simulink model "power_active_filter_mpc"  (R2019a)
settings: Solver=VariableStepAuto  StartTime=0.0  StopTime=1.5  RelTol=1e-3
values from neighbouring files (symbols this model uses):
  Ts = 2e-6    (= 2e-06)    [parameters.m]
  Vdc = AF.activefilter.voltage    [parameters.m]
undefined symbols (not defined in the file or in its folder): AF, D1, Delta, R
libraries: powerlib x28, powerlib_meascontrol x4, eeTransforms x3, dspstat3 x2, dsparch4 x2, simulink x1, eePwmGeneratorTwoLevel x1
settings Model: PauseTimes=0.51  Creator=Abdullah  LastModifiedBy=Abdullah
settings SolverCC: ShapePreserveControl=EnableAll  MinimalZcImpactIntegration=on
settings DataIOCC: SaveFormat=StructureWithTime  ReturnWorkspaceOutputs=off
settings DebuggingCC: ReadBeforeWriteMsg=DisableAll  WriteAfterWriteMsg=DisableAll  WriteAfterReadMsg=DisableAll  MultiTaskDSMMsg=none
settings ModelReferenceCC: UpdateModelReferenceTargets=IfOutOfDate
settings SFSimCC: SFSimEcho=off

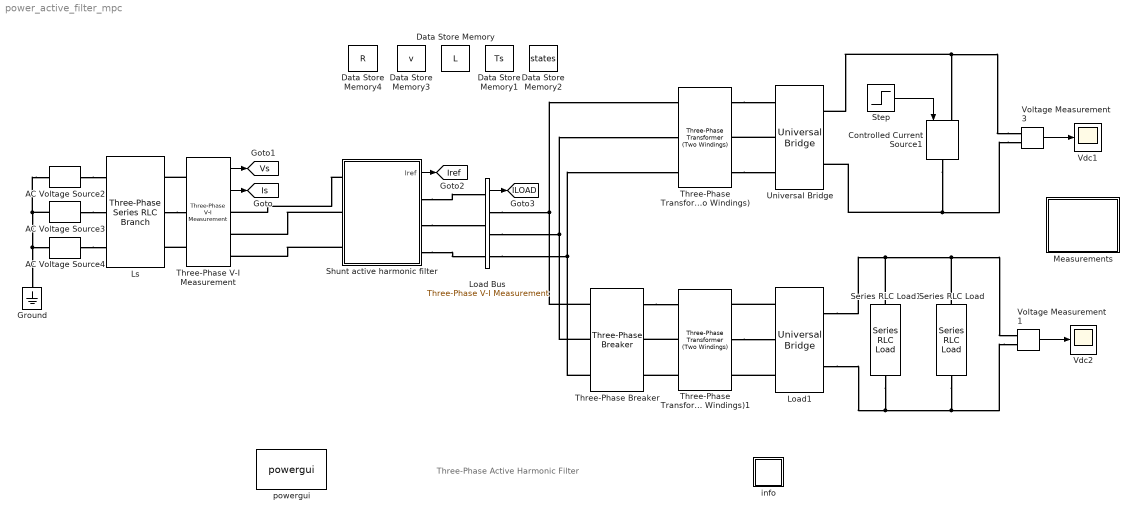
== system power_active_filter_mpc ==
  note: Three-Phase Active Harmonic Filter
  AC Voltage Source2 : powerlib/Electrical Sources/AC Voltage Source  Amplitude=380*sqrt(2)/sqrt(3)  Phase=0  Frequency=50  SampleTime=0  Measurements=None  BusType=swing  Pref=10e3  Qref=0  Qmin=-inf  Qmax=+inf
      settings: SourceProductName=Simscape Electrical
  AC Voltage Source3 : powerlib/Electrical Sources/AC Voltage Source  Amplitude=380*sqrt(2)/sqrt(3)  Phase=-120  Frequency=50  SampleTime=0  Measurements=None  BusType=swing  Pref=10e3  Qref=0  Qmin=-inf  Qmax=+inf
      settings: SourceProductName=Simscape Electrical
  AC Voltage Source4 : powerlib/Electrical Sources/AC Voltage Source  Amplitude=380*sqrt(2)/sqrt(3)  Phase=120  Frequency=50  SampleTime=0  Measurements=None  BusType=swing  Pref=10e3  Qref=0  Qmin=-inf  Qmax=+inf
      settings: SourceProductName=Simscape Electrical
  Controlled Current Source1 : powerlib/Electrical Sources/Controlled Current Source  Initialize=on  Source_Type=AC  Amplitude=0  Phase=0  Frequency=0  Measurements=None
      settings: SourceProductName=Simscape Electrical
  Data Store Memory : DataStoreMemory  DataStoreName=L  ReadBeforeWriteMsg=warning  WriteAfterWriteMsg=warning  WriteAfterReadMsg=warning  InitialValue=L  ShowAdditionalParam=off  OutDataTypeStr=double
  Data Store Memory1 : DataStoreMemory  DataStoreName=Ts  ReadBeforeWriteMsg=warning  WriteAfterWriteMsg=warning  WriteAfterReadMsg=warning  InitialValue=Ts  ShowAdditionalParam=off  OutDataTypeStr=double
  Data Store Memory2 : DataStoreMemory  DataStoreName=states  ReadBeforeWriteMsg=warning  WriteAfterWriteMsg=warning  WriteAfterReadMsg=warning  InitialValue=states  VectorParams1D=off  ShowAdditionalParam=off  OutDataTypeStr=double
  Data Store Memory3 : DataStoreMemory  DataStoreName=v  ReadBeforeWriteMsg=warning  WriteAfterWriteMsg=warning  WriteAfterReadMsg=warning  InitialValue=v  ShowAdditionalParam=off  OutDataTypeStr=double
      settings: SignalType=complex
  Data Store Memory4 : DataStoreMemory  DataStoreName=R  ReadBeforeWriteMsg=warning  WriteAfterWriteMsg=warning  WriteAfterReadMsg=warning  InitialValue=R  ShowAdditionalParam=off  OutDataTypeStr=double
  Ground : powerlib/Elements/Ground  LConnTagsString=a
      settings: SourceProductName=Simscape Electrical
  Load Bus : powerlib/Measurements/Three-Phase V-I Measurement  VoltageMeasurement=no  SetLabelV=off  LabelV=Vabc  Vpu=off  VpuLL=off  CurrentMeasurement=yes  SetLabelI=off  LabelI=ILoad  Ipu=off  Pbase=100e6  Vbase=500e3  OutputType=Complex  PhasorSimulation=off  PSBequivalent=0
      settings: SourceProductName=Simscape Electrical
  Load1 : powerlib/Power Electronics/Universal Bridge  Arms=3  SnubberResistance=1e3  SnubberCapacitance=1e-6  Device=Diodes  Ron=1e-3  Lon=0  ForwardVoltages="[  0  0  ]"  ForwardVoltage=0  GTOparameters=[ 10e-6 , 20e-6 ]  IGBTparameters=[ 1e-6 , 2e-6 ]  Measurements=None  Measurements_2=None  converterType=Rectifier
      settings: SourceProductName=Simscape Electrical
  Ls : powerlib/Elements/Three-Phase Series RLC Branch  LConnTagsString=A|B|C  RConnTagsString=A|B|C  BranchType=L  Resistance=1  Inductance=1e-5  Capacitance=1e-6  Measurements=None
      settings: SourceProductName=Simscape Electrical
  Measurements : Subsystem
  Series RLC Load : powerlib/Elements/Series RLC Load  LConnTagsString=a  RConnTagsString=__new0  NominalVoltage=500  NominalFrequency=50  ActivePower=50e3  InductivePower=10e3  CapacitivePower=0  Setx0=off  InitialVoltage=0  SetiL0=off  InitialCurrent=0  Measurements=None  LoadType=constant Z
      settings: SourceProductName=Simscape Electrical
  Series RLC Load1 : powerlib/Elements/Series RLC Load  LConnTagsString=a  RConnTagsString=__new0  NominalVoltage=500  NominalFrequency=50  ActivePower=0  InductivePower=0  CapacitivePower=20e3  Setx0=off  InitialVoltage=0  SetiL0=off  InitialCurrent=0  Measurements=None  LoadType=constant Z
      settings: SourceProductName=Simscape Electrical
  Shunt active harmonic filter : Subsystem  mask(Parallel Active Filter){platform=AF}
  Step : Step  Time=0.5  Before=100  After=160  SampleTime=0
  Three-Phase Transformer (Two Windings) : powerlib/Elements/Three-Phase Transformer (Two Windings)  Winding1Connection=Delta (D1)  Winding2Connection=Delta (D1)  CoreType=Three single-phase transformers  SetSaturation=off  Hysteresis=off  DataFile='hysteresis'  SetInitialFlux=off  Measurements=None  UNITS=pu  NominalPower=[ 500e3 , 50 ]  Winding1=[380, 0.002 , 0.08 ]  Winding2=[380, 0.002 , 0.08 ]  Rm=500  Lm=500  L0=0.5  Saturation=[ 0,0 ; 0.0024,1.2 ; 1.0,1.52 ]  InitialFluxes=[ 0.8 , -0.8 , 0.7 ]  BreakLoop=off  DiscreteSolver=Trapezoidal iterative  DataType=off  TransfoNumber=0
      settings: SourceProductName=Simscape Electrical
  Three-Phase Transformer (Two Windings)1 : powerlib/Elements/Three-Phase Transformer (Two Windings)  Winding1Connection=Delta (D1)  Winding2Connection=Y  CoreType=Three single-phase transformers  SetSaturation=off  Hysteresis=off  DataFile='hysteresis'  SetInitialFlux=off  Measurements=None  UNITS=pu  NominalPower=[ 500e3 , 50 ]  Winding1=[380, 0.002 , 0.08 ]  Winding2=[380, 0.002 , 0.08 ]  Rm=500  Lm=500  L0=0.5  Saturation=[ 0,0 ; 0.0024,1.2 ; 1.0,1.52 ]  InitialFluxes=[-0.000126716792896904 1.12530200800683e-05 0.000115463772816653]  BreakLoop=off  DiscreteSolver=Trapezoidal iterative  DataType=off  TransfoNumber=0
      settings: SourceProductName=Simscape Electrical
  Three-Phase V-I Measurement : powerlib/Measurements/Three-Phase V-I Measurement  VoltageMeasurement=phase-to-ground  SetLabelV=off  LabelV=Vabc  Vpu=off  VpuLL=off  CurrentMeasurement=yes  SetLabelI=off  LabelI=Iabc  Ipu=off  Pbase=100e6  Vbase=500e3  OutputType=Complex  PhasorSimulation=off  PSBequivalent=0
      settings: SourceProductName=Simscape Electrical
  Three-Phase Breaker : powerlib/Elements/Three-Phase Breaker  InitialState=open  SwitchA=on  SwitchB=on  SwitchC=on  SwitchTimes=1  External=off  BreakerResistance=1e-5  SnubberResistance=1e6  SnubberCapacitance=inf  Measurements=None
      settings: SourceProductName=Simscape Electrical
  Universal Bridge : powerlib/Power Electronics/Universal Bridge  Arms=3  SnubberResistance=1e5  SnubberCapacitance=inf  Device=Diodes  Ron=1e-3  Lon=0  ForwardVoltages="[  0  0  ]"  ForwardVoltage=0  GTOparameters=[ 10e-6 , 20e-6 ]  IGBTparameters=[ 1e-6 , 2e-6 ]  Measurements=None  Measurements_2=None  converterType=Rectifier
      settings: SourceProductName=Simscape Electrical
  Vdc1 : Scope
  Vdc2 : Scope
  Voltage Measurement1 : powerlib/Measurements/Voltage Measurement  PhasorSimulation=off  OutputType=Complex  PSBequivalent=0
      settings: SourceProductName=Simscape Electrical
  Voltage Measurement3 : powerlib/Measurements/Voltage Measurement  PhasorSimulation=off  OutputType=Complex  PSBequivalent=0
      settings: SourceProductName=Simscape Electrical
  info : Subsystem
      settings: OpenFcn=showdemo(bdroot(gcb))
      mask Display: disp('?')
  powergui : powerlib/powergui  SimulationMode=Discrete  SampleTime=Ts  frequency=60  Iterations=50  frequencyindice=0  Pbase=100e6  ErrMax=1e-4  UnitsV=kV  UnitsW=MW  buscounter=0  FunctionMessages=off  echomessages=off  EnableUseOfTLC=off  CurrentSourceSwitches=off  DisableSnubberDevices=off  DisableRonSwitches=off  DisableVfSwitches=off  DisplayEquations=off  AutomaticDiscreteSolvers=off  SolverType=Tustin/Backward Euler (TBE)  Interpol=off  ExternalGateDelay=off  methode=off  Ts=0  x0status=blocks  SPID=off  SwTol=0  HookPort=off  NonlinearTolerance=0  nMaxIteration=15  ContinueOnMaxIteration=off  RestoreLinks=warning  ResistiveCurrentMeasurement=off  Frange=[0:2:500]  Ylog=off  Xlog=on  ShowGrid=off  save=off  variable=ZData  structure=Filteroutput  ZoomFFT=off  StartTime=10/50  cycles=2  DisplayStyle=1  fundamental=50  FreqAxis=on  MaxFrequency=250000  frequencyindicesteady=1  RmsSteady=1  display=off
      settings: SourceProductName=Simscape Electrical
  tag scope: ILOAD=global, Iref=global, Is=global, Vs=global
  wires:
  Load Bus/1 -> [ILOAD]
  Three-Phase V-I Measurement/1 -> [Vs]
  Voltage Measurement3/1 -> Vdc1/1
  Shunt active harmonic filter/1(Iref) -> [Iref]
  Step/1 -> Controlled Current Source1/1
  Three-Phase V-I Measurement/2 -> [Is]
  Voltage Measurement1/1 -> Vdc2/1
  connections:
  Load Bus/RConn3 -- Three-Phase Breaker/LConn3 -- Three-Phase Transformer (Two Windings)/LConn3
  Load Bus/RConn1 -- Three-Phase Breaker/LConn1 -- Three-Phase Transformer (Two Windings)/LConn1
  Voltage Measurement3/LConn2 -- Universal Bridge/RConn2 -- Controlled Current Source1/RConn1
  AC Voltage Source2/LConn1 -- AC Voltage Source4/LConn1 -- Ground/LConn1 -- AC Voltage Source3/LConn1
  Load Bus/RConn2 -- Three-Phase Breaker/LConn2 -- Three-Phase Transformer (Two Windings)/LConn2
  Series RLC Load1/LConn1 -- Load1/RConn1 -- Series RLC Load/LConn1 -- Voltage Measurement1/LConn1
  Voltage Measurement1/LConn2 -- Series RLC Load/RConn1 -- Load1/RConn2 -- Series RLC Load1/RConn1
  Voltage Measurement3/LConn1 -- Universal Bridge/RConn1 -- Controlled Current Source1/LConn1
  AC Voltage Source4/RConn1 -- Ls/LConn3
  Shunt active harmonic filter/LConn3 -- Three-Phase V-I Measurement/RConn3
  Shunt active harmonic filter/LConn2 -- Three-Phase V-I Measurement/RConn2
  Three-Phase Transformer (Two Windings)/RConn1 -- Universal Bridge/LConn1
  Shunt active harmonic filter/RConn3 -- Load Bus/LConn3
  Shunt active harmonic filter/RConn1 -- Load Bus/LConn1
  Shunt active harmonic filter/RConn2 -- Load Bus/LConn2
  Shunt active harmonic filter/LConn1 -- Three-Phase V-I Measurement/RConn1
  Universal Bridge/LConn2 -- Three-Phase Transformer (Two Windings)/RConn2
  Three-Phase V-I Measurement/LConn1 -- Ls/RConn1
  Ls/RConn2 -- Three-Phase V-I Measurement/LConn2
  Three-Phase V-I Measurement/LConn3 -- Ls/RConn3
  AC Voltage Source2/RConn1 -- Ls/LConn1
  AC Voltage Source3/RConn1 -- Ls/LConn2
  Three-Phase Transformer (Two Windings)/RConn3 -- Universal Bridge/LConn3
  Load1/LConn1 -- Three-Phase Transformer (Two Windings)1/RConn1
  Three-Phase Transformer (Two Windings)1/RConn2 -- Load1/LConn2
  Load1/LConn3 -- Three-Phase Transformer (Two Windings)1/RConn3
  Three-Phase Breaker/RConn1 -- Three-Phase Transformer (Two Windings)1/LConn1
  Three-Phase Transformer (Two Windings)1/LConn2 -- Three-Phase Breaker/RConn2
  Three-Phase Transformer (Two Windings)1/LConn3 -- Three-Phase Breaker/RConn3

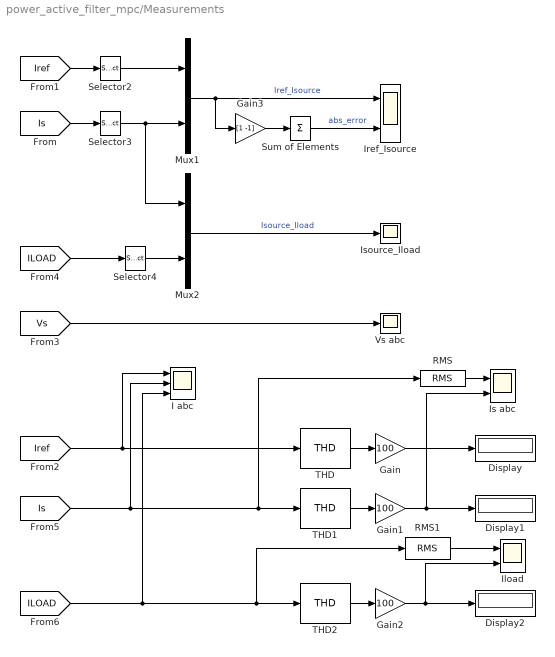
== system power_active_filter_mpc/Measurements ==
  Display : Display
  Display1 : Display
      settings: Decimation=2
  Display2 : Display
      settings: Decimation=2
  Gain : Gain  Gain=100
  Gain1 : Gain  Gain=100
  Gain2 : Gain  Gain=100
  Gain3 : Gain  Gain=[1 -1]
  I abc : Scope  NumInputPorts=3
  Iload : Scope  NumInputPorts=2
  Iref_Isource : Scope  NumInputPorts=2
  Is abc : Scope  NumInputPorts=2
  Isource_Iload : Scope
  Mux1 : Mux  Inputs=2
  Mux2 : Mux  Inputs=2
  RMS : dspstat3/RMS  run=off  directionMode=Each column  dimension=1  InputProcessing=Columns as channels (frame based)  reset_popup=None
  RMS1 : dspstat3/RMS  run=off  directionMode=Each column  dimension=1  InputProcessing=Columns as channels (frame based)  reset_popup=None
  Selector2 : Selector  InputPortWidth=3  IndexOptions=Index vector (dialog)  Indices=1  OutputSizes=1
  Selector3 : Selector  InputPortWidth=3  IndexOptions=Index vector (dialog)  Indices=1  OutputSizes=1
  Selector4 : Selector  InputPortWidth=3  IndexOptions=Index vector (dialog)  Indices=1  OutputSizes=1
  Sum of Elements : Sum  Inputs=+
  THD : powerlib_meascontrol/Measurements/THD  Freq=50  Ts=0
      settings: SourceProductName=Simscape Electrical
  THD1 : powerlib_meascontrol/Measurements/THD  Freq=50  Ts=0
      settings: SourceProductName=Simscape Electrical
  THD2 : powerlib_meascontrol/Measurements/THD  Freq=50  Ts=0
      settings: SourceProductName=Simscape Electrical
  Vs abc : Scope
  wires:
  Mux1/1 -> Gain3/1, Iref_Isource/1  "Iref_Isource"
  Selector2/1 -> Mux1/1
  Selector3/1 -> Mux1/2, Mux2/1
  [Iref] -> Selector2/1
  [Is] -> Selector3/1
  Mux2/1 -> Isource_Iload/1  "Isource_Iload"
  Selector4/1 -> Mux2/2
  [ILOAD] -> Selector4/1
  Gain3/1 -> Sum of Elements/1
  Sum of Elements/1 -> Iref_Isource/2  "abs_error"
  [Vs] -> Vs abc/1
  [Iref] -> THD/1, I abc/1
  [Is] -> RMS/1, THD1/1, I abc/2
  THD/1 -> Gain/1
  THD1/1 -> Gain1/1
  Gain/1 -> Display/1
  Gain1/1 -> Is abc/2, Display1/1
  THD2/1 -> Gain2/1
  RMS/1 -> Is abc/1
  RMS1/1 -> Iload/1
  Gain2/1 -> Iload/2, Display2/1
  [ILOAD] -> I abc/3, RMS1/1, THD2/1

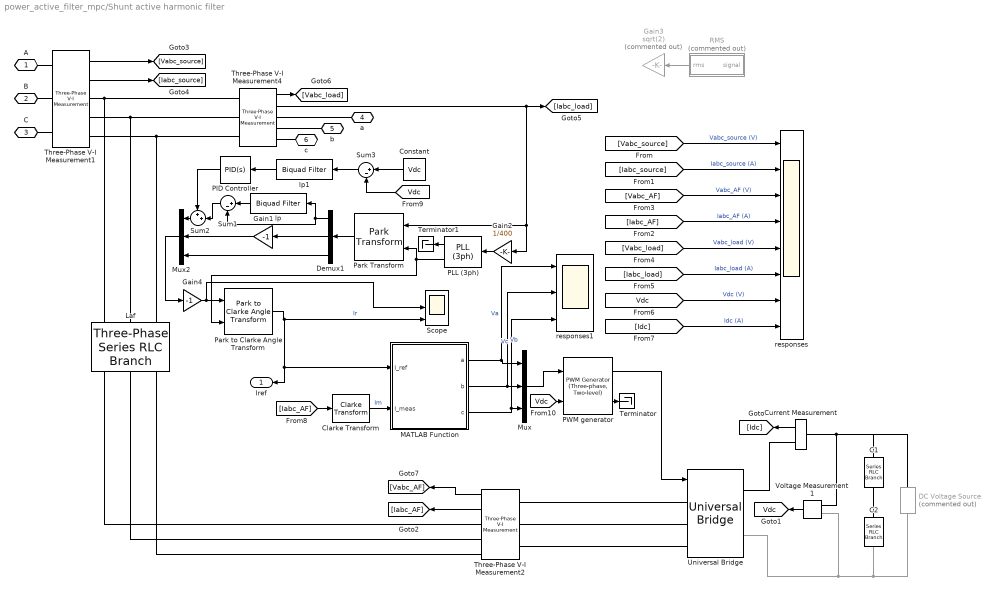
== system power_active_filter_mpc/Shunt active harmonic filter ==
  C1 : powerlib/Elements/Series RLC Branch  LConnTagsString=__new0  RConnTagsString=__new0  BranchType=C  Resistance=1  Inductance=1e-3  SetiL0=off  InitialCurrent=0  Capacitance=platform.activefilter.DC_cap  Setx0=on  InitialVoltage=Vdc/2  Measurements=None
      settings: SourceProductName=Simscape Electrical
  C2 : powerlib/Elements/Series RLC Branch  LConnTagsString=__new0  RConnTagsString=__new0  BranchType=C  Resistance=1  Inductance=1e-3  SetiL0=off  InitialCurrent=0  Capacitance=platform.activefilter.DC_cap  Setx0=on  InitialVoltage=Vdc/2  Measurements=None
      settings: SourceProductName=Simscape Electrical
  Clarke Transform : eeTransforms/Clarke Transform  PowerInvariant=off
      settings: SourceProductName=Simscape Electrical  SourceProductBaseCode=PS
  Constant : Constant  Value=Vdc
  Current Measurement : powerlib/Measurements/Current Measurement  PhasorSimulation=off  OutputType=Complex  PSBequivalent=0
      settings: SourceProductName=Simscape Electrical
  DC Voltage Source : powerlib/Electrical Sources/DC Voltage Source  Commented=on  Amplitude=Vdc  Measurements=None
      settings: SourceProductName=Simscape Electrical
  Demux1 : Demux  Outputs=3
  Gain1 : Gain  Gain=-1
  Gain2 : Gain  Gain=1/400
  Gain3 : Gain  Commented=on  Gain=sqrt(2)
  Gain4 : Gain  Gain=-1
  Laf : powerlib/Elements/Three-Phase Series RLC Branch  LConnTagsString=A|B|C  RConnTagsString=A|B|C  BranchType=RL  Resistance=R  Inductance=platform.activefilter.Laf  Capacitance=1e-6  Measurements=None
      settings: SourceProductName=Simscape Electrical
  MATLAB Function : MATLAB Function  TreatAsAtomicUnit=on  SystemSampleTime=Ts
  Mux : Mux  Inputs=3
  Mux2 : Mux  Inputs=3
  PID Controller : simulink/Continuous/PID Controller  Controller=PID  Form=Parallel  TimeDomain=Continuous-time  SampleTime=-1  IntegratorMethod=Forward Euler  FilterMethod=Forward Euler  ControllerParametersSource=internal  P=0.0255  I=0.75  D=0.0005  UseFilter=on  N=100  TunerSelectOption=Transfer Function Based (PID Tuner App)  InitialConditionSource=internal  InitialConditionForIntegrator=0  InitialConditionForFilter=0  DifferentiatorICPrevScaledInput=0  ExternalReset=none  TrackingMode=off  Kt=1  LimitOutput=off  UpperSaturationLimit=inf  LowerSaturationLimit=-inf  LinearizeAsGain=on  AntiWindupMode=none  Kb=1  POutMin=[]  POutMax=[]  IOutMin=[]  IOutMax=[]  DOutMin=[]  DOutMax=[]  NOutMin=[]  NOutMax=[]  SumOutMin=[]  SumOutMax=[]  SaturationOutMin=[]  SaturationOutMax=[]  PParamMin=[]  PParamMax=[]  IParamMin=[]  IParamMax=[]  DParamMin=[]  DParamMax=[]  NParamMin=[]  NParamMax=[]  KbParamMin=[]  KbParamMax=[]  KtParamMin=[]  KtParamMax=[]  KbOutMin=[]  KbOutMax=[]  KtOutMin=[]  KtOutMax=[]  IntegratorOutMin=[]  IntegratorOutMax=[]  FilterOutMin=[]  FilterOutMax=[]  SumI1OutMin=[]  SumI1OutMax=[]  SumI2OutMin=[]  SumI2OutMax=[]  SumI3OutMin=[]  SumI3OutMax=[]  SumI4OutMin=[]  SumI4OutMax=[]  SumDOutMin=[]  SumDOutMax=[]  DifferentiatorOutMin=[]  DifferentiatorOutMax=[]  FilterDiffOutCoefMin=[]  FilterDiffOutCoefMax=[]  ReciprocalOutMin=[]  ReciprocalOutMax=[]  SumDenOutMin=[]  SumDenOutMax=[]  SumNumOutMin=[]  SumNumOutMax=[]  DivideOutMin=[]  DivideOutMax=[]  IntegratorContinuousStateAttributes=''  IntegratorStateMustResolveToSignalObject=off  IntegratorRTWStateStorageClass=Auto  FilterContinuousStateAttributes=''  FilterStateMustResolveToSignalObject=off  FilterRTWStateStorageClass=Auto  ParallelPVariant=InternalParameters  IdealPVariant=Disabled  IVariant=InternalParameters  DVariant=InternalParameters  IntegratorVariant=Continuous  SatVariant=Disabled  AWVariant=Passthrough  PCopyVariant=Disabled  TRVariant=Disabled  FdbkBlocksVariant=Forward  IdealPFdbkVariant=Disabled  SatFdbkVariant=Disabled  DerivativeFilterVariant=ContFilter  NVariant=InternalParameters  NCopyVariant=Disabled  FilterICVariant=InternalICsFilter  IntegratorICVariant=InternalICs  ExternalResetVariant=Disabled  TRSumVariant=Passthrough  SumFdbkVariant=Disabled  SumVariant=Sum_PID
  PLL (3ph) : powerlib_meascontrol/PLL/PLL (3ph)  Fmin=45  Par_Init=[0 50]  ParK=[ 180 3200 1 ]  TcD=1e-3  MaxRateChangeFreq=12  FilterCutOffFreq=25  Ts=Ts  AGC=on
      settings: SourceProductName=Simscape Electrical
  PWM generator : eePwmGeneratorTwoLevel/PWM Generator (Three-phase, Two-level)  PWMMode=Continuous PWM (CPWM)  CPWMMode=SPWM: sinusoidal PWM  DPWMMode=60 DPWM: 60 degree discontinuous PWM  fsw=5000  Ts=Ts
      settings: SourceProductName=Simscape Electrical  SourceProductBaseCode=PS
  Park Transform : eeTransforms/Park Transform  AxisAlignment=Q-axis  PowerInvariant=off
      settings: SourceProductName=Simscape Electrical
  Park to Clarke Angle Transform : eeTransforms/Park to Clarke Angle Transform  AxisAlignment=Q-axis
      settings: SourceProductName=Simscape Electrical  SourceProductBaseCode=PS
  RMS : Subsystem  Commented=on  DialogController=POWERSYS.PowerSysDialog  mask(RMS){f1=platform.activefilter.freq}
      mask prompts: f1 "Fundamental frequency (Hz):"
      mask help: This block measures the root mean square value of instantaneous current or voltage signal connected to the input of the block. The RMS value is calculated over a running window of one cycle of the specified fundamental frequency.
      mask init:
      | power_initmask();
      mask Help: helpview(psbhelp)
  Scope : Scope  NumInputPorts=3
  Sum1 : Sum  Inputs=|+-
  Sum2 : Sum  Inputs=++|
  Sum3 : Sum  Inputs=|+-
  Terminator : Terminator
  Terminator1 : Terminator
  Three-Phase V-I Measurement1 : powerlib/Measurements/Three-Phase V-I Measurement  VoltageMeasurement=phase-to-phase  SetLabelV=off  LabelV=Vabc  Vpu=off  VpuLL=off  CurrentMeasurement=yes  SetLabelI=off  LabelI=Iabc  Ipu=off  Pbase=100e6  Vbase=500e3  OutputType=Complex  PhasorSimulation=off  PSBequivalent=0
      settings: SourceProductName=Simscape Electrical
  Three-Phase V-I Measurement2 : powerlib/Measurements/Three-Phase V-I Measurement  VoltageMeasurement=phase-to-phase  SetLabelV=off  LabelV=Vabc  Vpu=off  VpuLL=off  CurrentMeasurement=yes  SetLabelI=off  LabelI=Iabc  Ipu=off  Pbase=100e6  Vbase=500e3  OutputType=Complex  PhasorSimulation=off  PSBequivalent=0
      settings: SourceProductName=Simscape Electrical
  Three-Phase V-I Measurement4 : powerlib/Measurements/Three-Phase V-I Measurement  VoltageMeasurement=phase-to-phase  SetLabelV=off  LabelV=Vabc  Vpu=off  VpuLL=off  CurrentMeasurement=yes  SetLabelI=off  LabelI=Iabc  Ipu=off  Pbase=100e6  Vbase=500e3  OutputType=Complex  PhasorSimulation=off  PSBequivalent=0
      settings: SourceProductName=Simscape Electrical
  Universal Bridge : powerlib/Power Electronics/Universal Bridge  Arms=3  SnubberResistance=1e5  SnubberCapacitance=inf  Device=IGBT / Diodes  Ron=1e-3  Lon=0  ForwardVoltages="[  0  0  ]"  ForwardVoltage=0  GTOparameters=[ 10e-6 , 20e-6 ]  IGBTparameters=[ 1e-6 , 2e-6 ]  Measurements=None  Measurements_2=None  converterType=Rectifier
      settings: SourceProductName=Simscape Electrical
  Voltage Measurement1 : powerlib/Measurements/Voltage Measurement  PhasorSimulation=off  OutputType=Complex  PSBequivalent=0
      settings: SourceProductName=Simscape Electrical
  lp : dsparch4/Biquad Filter  Tag=BlockMethodSubSystem  FilterSource=Dialog parameters  CoeffSource=Specify via dialog  FilterObject=BQF  IIRFiltStruct=Direct form II  BiQuadCoeffs=[0.0548343892941136057 -0.109665070395729369 0.0548343892941136266 1 -1.99845906585976141 0.998464270664409792;1.00001025426045609 -2 1.00001025426045587 1 -1.99980794984853238 0.999822128007448074;0.00102649751294326286 0.00102649751294326286 0 1 -0.998953802933608026 0;1.00001336148623721 -2 1.00001336148623721 1 -1.99929745179046936 0.999308704544053739]  ScaleValues=[3.31889887857111711e-06;1;1;1;62738.3781479644313]  IC=0  ICnum=0  ICden=0  a0Flag=Warning  optimizeScaleValues=on  ScaleValueMode=Specify via input port (g)  roundingMode=Floor  overflowMode=off  scaleValueFracLength=14  denProdOutputFracLength=30  denAccumFracLength=30  secondMemoryFracLength=15
      settings: SourceProductName=DSP System Toolbox
  lp1 : dsparch4/Biquad Filter  Tag=BlockMethodSubSystem  FilterSource=Dialog parameters  CoeffSource=Specify via dialog  FilterObject=BQF  IIRFiltStruct=Direct form II  BiQuadCoeffs=[0.0548343892941136057 -0.109665070395729369 0.0548343892941136266 1 -1.99845906585976141 0.998464270664409792;1.00001025426045609 -2 1.00001025426045587 1 -1.99980794984853238 0.999822128007448074;0.00102649751294326286 0.00102649751294326286 0 1 -0.998953802933608026 0;1.00001336148623721 -2 1.00001336148623721 1 -1.99929745179046936 0.999308704544053739]  ScaleValues=[3.31889887857111711e-06;1;1;1;62738.3781479644313]  IC=0  ICnum=0  ICden=0  a0Flag=Warning  optimizeScaleValues=on  ScaleValueMode=Specify via input port (g)  roundingMode=Floor  overflowMode=off  scaleValueFracLength=14  denProdOutputFracLength=30  denAccumFracLength=30  secondMemoryFracLength=15
      settings: SourceProductName=DSP System Toolbox
  responses : Scope  NumInputPorts=8
  responses1 : Scope  NumInputPorts=3
  A : PMIOPort  Side=Left
  B : PMIOPort  Port=2  Side=Left
  C : PMIOPort  Port=3  Side=Left
  a : PMIOPort  Port=4  Side=Right
  b : PMIOPort  Port=5  Side=Right
  c : PMIOPort  Port=6  Side=Right
  Iref : Outport
  tag scope: Vdc=global
  wires:
  Three-Phase V-I Measurement2/2 -> [Iabc_AF]
  Current Measurement/1 -> [Idc]
  RMS/1(rms) -> Gain3/1
  Voltage Measurement1/1 -> [Vdc]
  Three-Phase V-I Measurement2/1 -> [Vabc_AF]
  Three-Phase V-I Measurement4/1 -> [Vabc_load]
  Three-Phase V-I Measurement1/1 -> [Vabc_source]
  Three-Phase V-I Measurement1/2 -> [Iabc_source]
  [Vabc_source] -> responses/1  "Vabc_source (V)"
  [Iabc_source] -> responses/2  "Iabc_source (A)"
  [Vabc_AF] -> responses/3  "Vabc_AF (V)"
  [Iabc_AF] -> responses/4  "Iabc_AF (A)"
  [Vabc_load] -> responses/5  "Vabc_load (V)"
  [Iabc_load] -> responses/6  "Iabc_load (A)"
  [Vdc] -> responses/7  "Vdc (V)"
  [Idc] -> responses/8  "Idc (A)"
  Clarke Transform/1 -> MATLAB Function/2(I_meas)  "Im"
  [Iabc_AF] -> Clarke Transform/1
  Gain2/1 -> PLL (3ph)/1
  PLL (3ph)/2 -> Park Transform/2, Park to Clarke Angle Transform/2
  Three-Phase V-I Measurement4/2 -> [Iabc_load], Park Transform/1, Gain2/1
  Park Transform/1 -> Demux1/1
  Demux1/1 -> Sum1/2, lp/1
  Demux1/3 -> Mux2/3
  lp/1 -> Sum1/1
  Demux1/2 -> Gain1/1
  Park to Clarke Angle Transform/1 -> Scope/3, MATLAB Function/1(I_ref), Iref/1  "Ir"
  Gain1/1 -> Mux2/2
  Gain4/1 -> Scope/2, Park to Clarke Angle Transform/1
  Mux2/1 -> Gain4/1
  Constant/1 -> Sum3/1
  [Vdc] -> Sum3/2
  Sum3/1 -> lp1/1
  lp1/1 -> PID Controller/1
  PID Controller/1 -> Sum2/1
  [Vdc] -> PWM generator/2
  Mux/1 -> PWM generator/1
  PWM generator/2 -> Terminator/1
  PLL (3ph)/1 -> Terminator1/1
  MATLAB Function/2(b) -> responses1/2, Mux/2  "Vb"
  MATLAB Function/1(a) -> responses1/1, Mux/1  "Va"
  MATLAB Function/3(c) -> responses1/3, Mux/3  "Vc"
  PWM generator/1 -> Universal Bridge/1
  Sum2/1 -> Mux2/1
  Sum1/1 -> Sum2/2
  connections:
  Voltage Measurement1/LConn1 -- C1/LConn1 -- DC Voltage Source/RConn1 -- Current Measurement/LConn1
  C2/LConn1 -- C1/RConn1
  DC Voltage Source/LConn1 -- C2/RConn1 -- Universal Bridge/RConn2 -- Voltage Measurement1/LConn2
  Universal Bridge/RConn1 -- Current Measurement/RConn1
  Three-Phase V-I Measurement1/RConn1 -- Three-Phase V-I Measurement4/LConn1 -- Laf/RConn1
  Three-Phase V-I Measurement1/RConn2 -- Three-Phase V-I Measurement4/LConn2 -- Laf/RConn2
  Three-Phase V-I Measurement1/RConn3 -- Three-Phase V-I Measurement4/LConn3 -- Laf/RConn3
  a/RConn1 -- Three-Phase V-I Measurement4/RConn1
  b/RConn1 -- Three-Phase V-I Measurement4/RConn2
  c/RConn1 -- Three-Phase V-I Measurement4/RConn3
  C/RConn1 -- Three-Phase V-I Measurement1/LConn3
  Three-Phase V-I Measurement1/LConn2 -- B/RConn1
  A/RConn1 -- Three-Phase V-I Measurement1/LConn1
  Three-Phase V-I Measurement2/LConn2 -- Universal Bridge/LConn2
  Universal Bridge/LConn1 -- Three-Phase V-I Measurement2/LConn1
  Three-Phase V-I Measurement2/LConn3 -- Universal Bridge/LConn3
  Three-Phase V-I Measurement2/RConn3 -- Laf/LConn3
  Three-Phase V-I Measurement2/RConn2 -- Laf/LConn2
  Three-Phase V-I Measurement2/RConn1 -- Laf/LConn1

== system power_active_filter_mpc/info ==

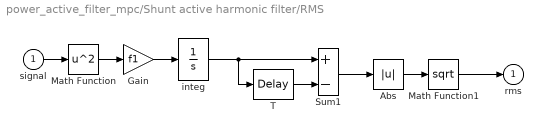
== system power_active_filter_mpc/Shunt active harmonic filter/RMS ==
  signal : Inport
  Abs : Abs  SaturateOnIntegerOverflow=on
  Gain : Gain  Gain=f1  SaturateOnIntegerOverflow=on  OutDataTypeStr=Inherit: Same as input  ParamDataTypeStr=Inherit: Same as input
  Math Function : Math  Operator=square  SaturateOnIntegerOverflow=on
  Math Function1 : Math  Operator=sqrt  SaturateOnIntegerOverflow=on
  Sum1 : Sum  Inputs=+-  SaturateOnIntegerOverflow=on  InputSameDT=on  OutDataTypeStr=Inherit: Same as first input
  T : TransportDelay  DelayTime=1/f1  BufferSize=9216
  integ : Integrator
  rms : Outport  InitialOutput=0
  wires:
  Gain/1 -> integ/1
  Math Function/1 -> Gain/1
  signal/1 -> Math Function/1
  Math Function1/1 -> rms/1
  integ/1 -> Sum1/1, T/1
  T/1 -> Sum1/2
  Sum1/1 -> Abs/1
  Abs/1 -> Math Function1/1

== matlab function power_active_filter_mpc/Shunt active harmonic filter/MATLAB Function ==
  settings: updateMethod=DISCRETE  sampleTime=Ts
  data: I_ref input; a output; I_meas input; b output; c output; Ts data_store_memory; L data_store_memory; v data_store_memory; states data_store_memory; R data_store_memory
function [a,b,c] = control(I_ref,I_meas)%,Vs)
% Variables defined in the parameters file
global Ts L R
% Optimum vector and measured current at instant k-1
persistent v_old i_old

K = Ts/L;

% Initialize values
if isempty(v_old), v_old = 0+1j*0; end
if isempty(i_old), i_old = 0+1j*0; end
% g_opt = 1e10;
% x_opt = 1;
% Read current reference inputs at sampling instant k
ik_ref = I_ref(1) + 1j*I_ref(2);
% Read current measurements at sampling instant k
ik = I_meas(1) + 1j*I_meas(2);

epsilon = 1e-2;
i=0;
g_opt = 1e10;
v_o1 = 0+0i;
alpha = 800;
e=1e5 + 1e5*1j;

% Vs_est = Vs(1) + 1j*Vs(2);
Vs_est = (L/Ts-R)*i_old + v_old - L/Ts*ik;

ik1 = K*v_o1 - K*Vs_est + (1-R*K)*ik;
% initial cost
g = (ik_ref - ik1)^2;
grad_g = -2*K*(ik_ref - (K*v_o1 - K*Vs_est + (1-R*K)*ik));

% Store the measured current for the next iteration
i_old = ik;

while e > epsilon
    
    grad_g = -2*K*(ik_ref - (K*v_o1 - K*Vs_est + (1-R*K)*ik));
    v_o1 = v_o1 - alpha * grad_g;
    
    ik1 = K*v_o1 - K*Vs_est + (1-R*K)*ik;
    g_opt = (ik_ref - ik1)^2; 

    e = g - g_opt;
    i = i+1;
    g = g_opt;

end
v_old = v_o1;
g = (ik_ref - ik1)^2;
g = (ik_ref - ik1)^2;

Alpha = real(v_o1);
Beta = imag(v_o1);
Zero = 0;

a = (Alpha + (0 .* Beta) + Zero);
b = (((-1/2) .* Alpha) + ((sqrt(3)/2) .* Beta) + ((1) .* Zero));
c = (((-1/2) .* Alpha) - ((sqrt(3)/2) .* Beta) + ((1) .* Zero));
